simulink model "msfcndemo_timestwo"  (Simulink 7.6)
settings: Solver=FixedStepDiscrete  StartTime=0.0  StopTime=10.0  RelTol=1e-3
settings Model: Creator=The MathWorks Inc.  ExtModeTrigMode=oneshot  ExtModeArmWhenConnect=off  ExtModeAutoUpdateStatusClock=off
settings DataIOCC: LimitDataPoints=off
settings OptimizationCC: BooleanDataType=off  InlineInvariantSignals=on  InitFltsAndDblsToZero=on
settings DebuggingCC: SaveWithParameterizedLinksMsg=none  SignalResolutionControl=TryResolveAllWithWarning  SolverPrmCheckMsg=none  MultiTaskDSMMsg=warning  MultiTaskCondExecSysMsg=none
settings HardwareCC: TargetUnknown=on
settings RTWCC: IncludeERTFirstTime=on
settings GRTTargetCC: TargetFcnLib=ansi_tfl_tmw.mat

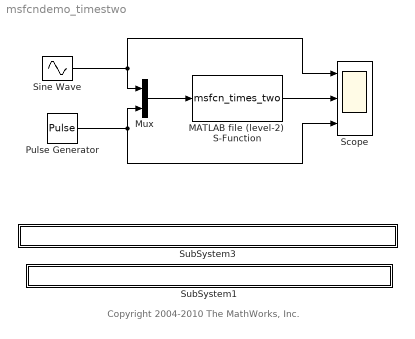
== system msfcndemo_timestwo ==
  note: Copyright 2004-2010 The MathWorks, Inc.
  MATLAB file (level-2)  S-Function : M-S-Function  FunctionName=msfcn_times_two
      mask Type: S-function: msfcn_times_two
      mask Description: This is a level-2 MATLAB file S-function which multiply input by two.
      mask Display:
      | plot([0 1 2 3 4 5 6 5 4 3 2 1 0 0],[0 .5 1 1.5 2 2.5 3 3.5 4 4.5 5 5.5 6 0]);
      | disp('2      ');
  Mux : Mux  Inputs=2
  Pulse Generator : DiscretePulseGenerator  PulseType=Time based  Amplitude=1:3  Period=1  PulseWidth=50
  Scope : Scope  NumInputPorts=3
      settings: TimeRange=10  YMin=-2~-5~0  YMax=2~10~3
  Sine Wave : Sin  Amplitude=1:2  SampleTime=0
  SubSystem1 : Subsystem  mask{filename=msfcn_times_two.m}
      mask init:
      | x=sfundemo_maskdisp;
      settings: AttributesFormatString=\n  OpenFcn=sfundemo_openfcn
      mask Display: disp(x);
  SubSystem3 : Subsystem  mask{filename=msfcn_times_two.tlc}
      mask init:
      | x=sfundemo_maskdisp;
      settings: AttributesFormatString=\n  OpenFcn=sfundemo_openfcn
      mask Display: disp(x);
  wires:
  MATLAB file (level-2)  S-Function/1 -> Scope/2
  Mux/1 -> MATLAB file (level-2)  S-Function/1
  Pulse Generator/1 -> Mux/2, Scope/3
  Sine Wave/1 -> Mux/1, Scope/1

== system msfcndemo_timestwo/SubSystem1 ==

== system msfcndemo_timestwo/SubSystem3 ==
